simulink library "tqd"  (R2021b)
settings: Solver=VariableStepAuto  StartTime=0.0  StopTime=10.0  RelTol=1e-3
undefined symbols (not defined in the file or in its folder): ATQD_BOSEnBPSPosn_X_kph, ATQD_BOSMap_X_rpm, ATQD_BOSMap_Y_pct, ATQD_CreepBaseTqD_X_kph, ATQD_CreepBaseTqD_Y_Deg, ATQD_CreepBaseTqR_X_kph, ATQD_CreepBaseTqR_Y_Deg, ATQD_CreepBPSDisPosn_X_Deg, ATQD_CreepBPSDisPosnR_X_Deg, ATQD_CreepBPSEnPosn_X_Deg, ATQD_CreepBPSEnPosnR_X_Deg, ATQD_CreepDeltaTq_X_kph, ATQD_CreepIterm_X_kph, ATQD_CreepIterm_Y_kph, ATQD_CreepItermMaxLimit_X_pct, ATQD_CreepPreloadTime_X_kph, ATQD_CreepPreloadTq_X_kph, ATQD_CreepPreloadTq_Y_s, ATQD_CreepProtTq_X_Deg, ATQD_CreepPterm_X_kph, ATQD_ECOTqMapD_X_rpm, ATQD_ECOTqMapD_Y_pct, ATQD_NL1TqMapD_X_rpm, ATQD_NL1TqMapD_Y_pct, ATQD_NRMRrEDUSpRat_X_rpm, ATQD_NRMRrEDUSpRat_Y_Nm, ATQD_PedalMapClimbUpLim_X_rpm, ATQD_PedalMapClimbUpLim_Y_Deg, ATQD_PreLoadTq_X_s, ATQD_SL1TqMapD_X_rpm, ATQD_SL1TqMapD_Y_pct, ATQD_WhlTqCapMotGain_X_pct, ATQD_WhlTqCapMotGain_Y_mV, ENUM_ACCPEDALLOWSW_LOWIDLE, ENUM_ACCPEDALLOWSW_NOIDLE, ENUM_CHRGPLUGSTA_NONE, ENUM_CRASHSTATE_NOCRASH, ENUM_DCDCFAULTSTA_WORKING, ENUM_DRIVEMODE_ECO, ENUM_DRIVEMODE_NRM, ENUM_DRIVEMODE_SPORT, ENUM_DRIVETRAIN_AWD, ENUM_DRIVETRAIN_FWD, ENUM_DRIVETRAIN_RWD, ENUM_EBSBRKSW_PRESSED, ENUM_EBSTORQUERWQ_LIMIT, ENUM_EBSTORQUERWQ_TORQUE, ENUM_EMTRQMODE_ACCL, ENUM_EMTRQMODE_BRAKING, ENUM_EMTRQMODE_COASTING, ENUM_EPBERROR_NORMAL, ENUM_EPBSTA_APPLIED, ENUM_EPBSTA_RELEASED, ENUM_EPBSTA_UNKNOWN, ENUM_EPBSTARAW_NOTSET, ENUM_EPBSTARAW_SET, ENUM_GEARACTUALPOSN_D, ENUM_GEARACTUALPOSN_N, ENUM_GEARACTUALPOSN_P, ENUM_GEARACTUALPOSN_R ... (+201)
libraries: hcu_lib x19, simulink x12
(part 5 of 6)

== system tqd/TQD/TorqueDemand/TorqueModule/AvaliableTqLimit/TorqueCapacityCalcalation ==
  VTQD_FrShaftSpd_rpm : Inport
  VTQD_RrShaftSpd_rpm : Inport  Port=2
  VINP_HVBPwrAvailDchrg_kw : Inport  Port=3
  VINP_HVBPwrAvailChrg_kw : Inport  Port=4
  KTQD_FrBatapCont_factor : Inport  Port=5
  KTQD_RrBatapCont_factor : Inport  Port=6
  VTQD_FrEDUSpRat_cmd : Inport  Port=7
  VTQD_RrEDUSpRat_rat : Inport  Port=8
  VINP_HVBCellVoltMax_mV : Inport  Port=9
  VINP_HVBCellVoltMin_mV : Inport  Port=10
  VINP_HVBSOH_pct : Inport  Port=11
  VTQD_GearActualPosn_enum : Inport  Port=12
  CapacityDistribution : Subsystem
  Constant19 : Constant  Value=MINUSONE_FLOAT
  Constant2 : Constant  Value=ENUM_GEARACTUALPOSN_R
  Data Type Conversion{,1..3} (4 alike) : DataTypeConversion  OutDataTypeStr=single
  Demux : Demux
  Equal : RelationalOperator  Operator===  OutDataTypeStr=boolean  RndMeth=Simplest
  Generation : Subsystem
  Motoring : Subsystem
  Mux : Mux
  Mux1 : Mux
  Product : Product
  Switch : Switch  Criteria=u2 > Threshold
  TMAvailablePwr_Calculation : Subsystem
  VTQD_WhlTqCapGenFr_Nm : Outport
  VTQD_WhlTqCapGenRr_Nm : Outport  Port=2
  VTQD_ActTqCapPosFr_Nm : Outport  Port=3
  VTQD_ActTqCapPosRr_Nm : Outport  Port=4
  VTQD_ActTqCapNegFr_Nm : Outport  Port=5
  VTQD_ActTqCapNegRr_Nm : Outport  Port=6
  wires:
  [VTQD_TMPwrAvailDchrg_kW] -> CapacityDistribution/3(VTQD_TMPwrAvailDchrg_kW)
  TMAvailablePwr_Calculation/1(VTQD_TMPwrAvailDchrg_kW) -> [VTQD_TMPwrAvailDchrg_kW]
  [VINP_HVBPwrAvailDchrg_kw] -> TMAvailablePwr_Calculation/1(VINP_HVBPwrAvailDchrg_kw)
  Motoring/2(VTQD_WhlTqCapMotRr_Nm) -> [VTQD_WhlTqCapMotRr_Nm]
  [VTQD_RrEDUSpRat_rat] -> CapacityDistribution/2(VTQD_RrEDUSpRat_rat)
  [VTQD_FrEDUSpRat_rat] -> CapacityDistribution/1(VTQD_FrEDUSpRat_cmd)
  CapacityDistribution/4(VTQD_RrHVBPwrAvailChrg_kw) -> [VTQD_RrHVBPwrAvailChrg_kw]
  CapacityDistribution/3(VTQD_FrHVBPwrAvailChrg_kw) -> [VTQD_FrHVBPwrAvailChrg_kw]
  CapacityDistribution/2(VTQD_RrHVBPwrAvailDchrg_kw) -> [VTQD_RrHVBPwrAvailDchrg_kw]
  CapacityDistribution/1(VTQD_FrHVBPwrAvailDchrg_kw) -> [VTQD_FrHVBPwrAvailDchrg_kw]
  [VINP_HVBPwrAvailChrg_kw] -> CapacityDistribution/4(VINP_HVBPwrAvailChrg_kw)
  [VTQD_RrHVBPwrAvailChrg_kw] -> Generation/4(VTQD_RrHVBPwrAvailChrg_kw)
  [KTQD_RrBatapCont_factor] -> Generation/6(KTQD_RrBatapCont_factor)
  [VTQD_FrShaftSpd_rpm] -> Generation/1(VTQD_FrShaftSpd_rpm)
  [VTQD_FrHVBPwrAvailChrg_kw] -> Generation/3(VTQD_FrHVBPwrAvailChrg_kw)
  [VTQD_RrShaftSpd_rpm] -> Generation/2(VTQD_RrShaftSpd_rpm)
  [KTQD_FrBatapCont_factor] -> Generation/5(KTQD_FrBatapCont_factor)
  Generation/1(VTQD_WhlTqCapGenFr_Nm) -> [VTQD_WhlTqCapGenFr_Nm], VTQD_WhlTqCapGenFr_Nm/1
  Generation/2(VTQD_WhlTqCapGenRr_Nm) -> [VTQD_WhlTqCapGenRr_Nm], VTQD_WhlTqCapGenRr_Nm/1
  [VTQD_RrHVBPwrAvailDchrg_kw] -> Motoring/4(VTQD_RrHVBPwrAvailDchrg_kw)
  [VTQD_FrHVBPwrAvailDchrg_kw] -> Motoring/3(VTQD_FrHVBPwrAvailDchrg_kw)
  [KTQD_RrBatapCont_factor] -> Motoring/6(KTQD_RrBatapCont_factor)
  VTQD_RrEDUSpRat_rat/1 -> [VTQD_RrEDUSpRat_rat]
  VTQD_FrEDUSpRat_cmd/1 -> [VTQD_FrEDUSpRat_rat]
  KTQD_RrBatapCont_factor/1 -> [KTQD_RrBatapCont_factor]
  [VTQD_RrShaftSpd_rpm] -> Motoring/2(VTQD_RrShaftSpd_rpm)
  VTQD_RrShaftSpd_rpm/1 -> [VTQD_RrShaftSpd_rpm]
  VTQD_FrShaftSpd_rpm/1 -> [VTQD_FrShaftSpd_rpm]
  VINP_HVBPwrAvailChrg_kw/1 -> [VINP_HVBPwrAvailChrg_kw]
  VINP_HVBPwrAvailDchrg_kw/1 -> [VINP_HVBPwrAvailDchrg_kw]
  KTQD_FrBatapCont_factor/1 -> [KTQD_FrBatapCont_factor]
  [VTQD_FrShaftSpd_rpm] -> Motoring/1(VTQD_FrShaftSpd_rpm)
  Motoring/1(VTQD_WhlTqCapMotFr_Nm) -> [VTQD_WhlTqCapMotFr_Nm]
  [KTQD_FrBatapCont_factor] -> Motoring/5(KTQD_FrBatapCont_factor)
  VINP_HVBSOH_pct/1 -> [VINP_HVBSOH_pct]
  VINP_HVBCellVoltMin_mV/1 -> [VINP_HVBCellVoltMin_mV]
  VINP_HVBCellVoltMax_mV/1 -> [VINP_HVBCellVoltMax_mV]
  [VINP_HVBSOH_pct] -> Motoring/9(VINP_HVBSOH_pct)
  [VINP_HVBCellVoltMin_mV] -> Motoring/8(VINP_HVBCellVoltMin_mV)
  [VINP_HVBCellVoltMax_mV] -> Motoring/7(VINP_HVBCellVoltMax_mV)
  VTQD_GearActualPosn_enum/1 -> [VTQD_GearActualPosn_enum]
  [VTQD_GearActualPosn_enum] -> Equal/1
  Constant2/1 -> Equal/2
  Equal/1 -> Switch/2
  Mux/1 -> Product/1
  Product/1 -> Switch/1
  Constant19/1 -> Product/2
  Mux1/1 -> Switch/3
  [VTQD_WhlTqCapMotFr_Nm] -> Mux1/1
  [VTQD_WhlTqCapMotRr_Nm] -> Mux1/2
  [VTQD_WhlTqCapGenFr_Nm] -> Mux1/3
  [VTQD_WhlTqCapGenRr_Nm] -> Mux1/4
  Switch/1 -> Demux/1
  [VTQD_WhlTqCapGenFr_Nm] -> Mux/1
  [VTQD_WhlTqCapGenRr_Nm] -> Mux/2
  [VTQD_WhlTqCapMotFr_Nm] -> Mux/3
  [VTQD_WhlTqCapMotRr_Nm] -> Mux/4
  Demux/1 -> Data Type Conversion/1
  Data Type Conversion/1 -> VTQD_ActTqCapPosFr_Nm/1  "VTQD_ActTqCapPosFr_Nm"
  Demux/2 -> Data Type Conversion1/1
  Data Type Conversion1/1 -> VTQD_ActTqCapPosRr_Nm/1  "VTQD_ActTqCapPosRr_Nm"
  Demux/3 -> Data Type Conversion2/1
  Data Type Conversion2/1 -> VTQD_ActTqCapNegFr_Nm/1  "VTQD_ActTqCapNegFr_Nm"
  Demux/4 -> Data Type Conversion3/1
  Data Type Conversion3/1 -> VTQD_ActTqCapNegRr_Nm/1  "VTQD_ActTqCapNegRr_Nm"

== system tqd/TQD/TorqueDemand/TorqueModule/DriverWhlTqDem/BOS ==
  VTQD_ActBPSPosn_pct : Inport
  VTQD_TqTargetShaftSpd_rpm : Inport  Port=2
  VTQD_VehActSpd_kph : Inport  Port=3
  VTQD_PedalMapWhlTq_Nm : Inport  Port=4
  VTQD_CreepBaseTqR_Nm : Inport  Port=5
  VTQD_CreepBaseTqD_Nm : Inport  Port=6
  VTQD_GearActualPosn_enum : Inport  Port=7
  VTQD_LowIdleAccPedal_flg : Inport  Port=8
  VTQD_HighBPSPosn_flg : Inport  Port=9
  VTQD_BrkSwSta_flg : Inport  Port=10
  AND : Logic  Inputs=3  AllPortsSameDT=off  OutDataTypeStr=boolean
  AND1 : Logic  AllPortsSameDT=off  OutDataTypeStr=boolean
  AND2 : Logic  AllPortsSameDT=off  OutDataTypeStr=boolean
  Constant1 : Constant  Value=KTQD_BOSEnPedalTq_Nm
  Constant18 : Constant  Value=ZERO_FLOAT
  Constant20 : Constant  Value=ENUM_GEARACTUALPOSN_R
  Constant3 : Constant  Value=ONE_PERCENT
  Detect Change : simulink/Logic and Bit Operations/Detect Change  vinit=0  OutDataTypeStr=boolean
  Equal10 : RelationalOperator  Operator===  OutDataTypeStr=boolean  RndMeth=Simplest
  MTQD_BOSEnBPSPosn_Y_pct : Lookup_n-D  NumberOfTableDimensions=1  BreakpointsForDimension1=ATQD_BOSEnBPSPosn_X_kph  Table=MTQD_BOSEnBPSPosn_Y_pct  InternalRulePriority=Speed  RndMeth=Simplest  InputSameDT=on
  MTQD_BOSMap_Z_pct : Lookup_n-D  BreakpointsForDimension1=ATQD_BOSMap_Y_pct  BreakpointsForDimension2=ATQD_BOSMap_X_rpm  Table=MTQD_BOSMap_Z_pct  ExtrapMethod=Clip  InternalRulePriority=Speed  RndMeth=Simplest  InputSameDT=on
      settings: InputPortMap=u0,u1
  Max : MinMax  Function=max  Inputs=2
  NOT1 : Logic  Operator=NOT  AllPortsSameDT=off  OutDataTypeStr=boolean
  NOT2 : Logic  Operator=NOT  AllPortsSameDT=off  OutDataTypeStr=boolean
  NOT3 : Logic  Operator=NOT  AllPortsSameDT=off  OutDataTypeStr=boolean
  OR : Logic  Operator=OR  Inputs=3  AllPortsSameDT=off  OutDataTypeStr=boolean
  OR1 : Logic  Operator=OR  AllPortsSameDT=off  OutDataTypeStr=boolean
  Product1 : Product  RndMeth=Zero
  Product2 : Product  RndMeth=Zero
  Product3 : Product  RndMeth=Zero
  Relational Operator : RelationalOperator  Operator=>  OutDataTypeStr=boolean  RndMeth=Simplest
  Relational Operator1 : RelationalOperator  Operator=>  OutDataTypeStr=boolean  RndMeth=Simplest
  Relational Operator2 : RelationalOperator  OutDataTypeStr=boolean  RndMeth=Simplest
  Relational Operator5 : RelationalOperator  Operator=>  OutDataTypeStr=boolean  RndMeth=Simplest
  SR_Latch : hcu_lib/Basic_Blocks/SR_Latch
  Switch7 : Switch  Criteria=u2 > Threshold
  Switch8 : Switch  Criteria=u2 > Threshold
  VTQD_BOSEnable_flg : Outport
  VTQD_BOSTq_Nm : Outport  Port=2
  wires:
  VTQD_TqTargetShaftSpd_rpm/1 -> [VTQD_TqTargetShaftSpd_rpm]
  [VTQD_ActBPSPosn_pct] -> MTQD_BOSMap_Z_pct/1
  [VTQD_TqTargetShaftSpd_rpm] -> MTQD_BOSMap_Z_pct/2
  Constant3/1 -> Product1/2
  Product1/1 -> [VTQD_BOSReduction_gain]  "VTQD_BOSReduction_gain"
  MTQD_BOSMap_Z_pct/1 -> Product1/1
  VTQD_ActBPSPosn_pct/1 -> [VTQD_ActBPSPosn_pct]
  Relational Operator/1 -> AND/1
  VTQD_VehActSpd_kph/1 -> [VTQD_VehActSpd_kph]
  [VTQD_VehActSpd_kph] -> MTQD_BOSEnBPSPosn_Y_pct/1
  MTQD_BOSEnBPSPosn_Y_pct/1 -> Relational Operator/2  "VTQD_BOSEnBPSPosn_pct"
  [VTQD_ActBPSPosn_pct] -> Relational Operator/1
  VTQD_PedalMapWhlTq_Nm/1 -> [VTQD_PedalMapWhlTq_Nm]
  Relational Operator1/1 -> AND/2
  [VTQD_PedalMapWhlTq_Nm] -> Relational Operator1/1
  Constant1/1 -> Relational Operator1/2
  [VTQD_PedalMapWhlTq_Nm] -> Product2/1
  [VTQD_BOSReduction_gain] -> Product2/2
  Product3/1 -> Max/2
  Switch8/1 -> VTQD_BOSTq_Nm/1, [VTQD_BOSTq_Nm]  "VTQD_BOSTq_Nm"
  [VTQD_CreepBaseTqR_Nm] -> Switch7/1
  Max/1 -> Switch8/1
  Product2/1 -> Switch8/3
  Equal10/1 -> Switch7/2
  [VTQD_PedalMapWhlTq_Nm] -> Product3/1
  [VTQD_BOSReduction_gain] -> Product3/2
  [VTQD_GearActualPosn_enum] -> Equal10/1
  Relational Operator5/1 -> Switch8/2
  Constant20/1 -> Equal10/2
  Switch7/1 -> Max/1
  Constant18/1 -> Relational Operator5/2
  [VTQD_CreepBaseTqD_Nm] -> Switch7/3
  VTQD_CreepBaseTqD_Nm/1 -> [VTQD_CreepBaseTqD_Nm]
  VTQD_CreepBaseTqR_Nm/1 -> [VTQD_CreepBaseTqR_Nm]
  VTQD_GearActualPosn_enum/1 -> [VTQD_GearActualPosn_enum]
  [VTQD_BOSReduction_gain] -> Relational Operator5/1
  AND/1 -> SR_Latch/1, NOT1/1
  SR_Latch/1 -> VTQD_BOSEnable_flg/1  "VTQD_BOSEnable_flg"
  NOT1/1 -> AND1/1
  [VTQD_BOSTq_Nm] -> Relational Operator2/2
  [VTQD_PedalMapWhlTq_Nm] -> Relational Operator2/1
  VTQD_LowIdleAccPedal_flg/1 -> [VTQD_LowIdleAccPedal_flg]
  [VTQD_LowIdleAccPedal_flg] -> NOT2/1
  NOT2/1 -> AND/3
  [VTQD_BrkSwSta_flg] -> NOT3/1
  AND2/1 -> OR/3
  [VTQD_GearActualPosn_enum] -> Detect Change/1
  [VTQD_HighBPSPosn_flg] -> OR/2
  NOT3/1 -> AND2/2
  [VTQD_LowIdleAccPedal_flg] -> AND2/1
  OR/1 -> AND1/2
  Detect Change/1 -> OR1/2
  Relational Operator2/1 -> OR/1
  AND1/1 -> OR1/1
  OR1/1 -> SR_Latch/2
  VTQD_BrkSwSta_flg/1 -> [VTQD_BrkSwSta_flg]
  VTQD_HighBPSPosn_flg/1 -> [VTQD_HighBPSPosn_flg]

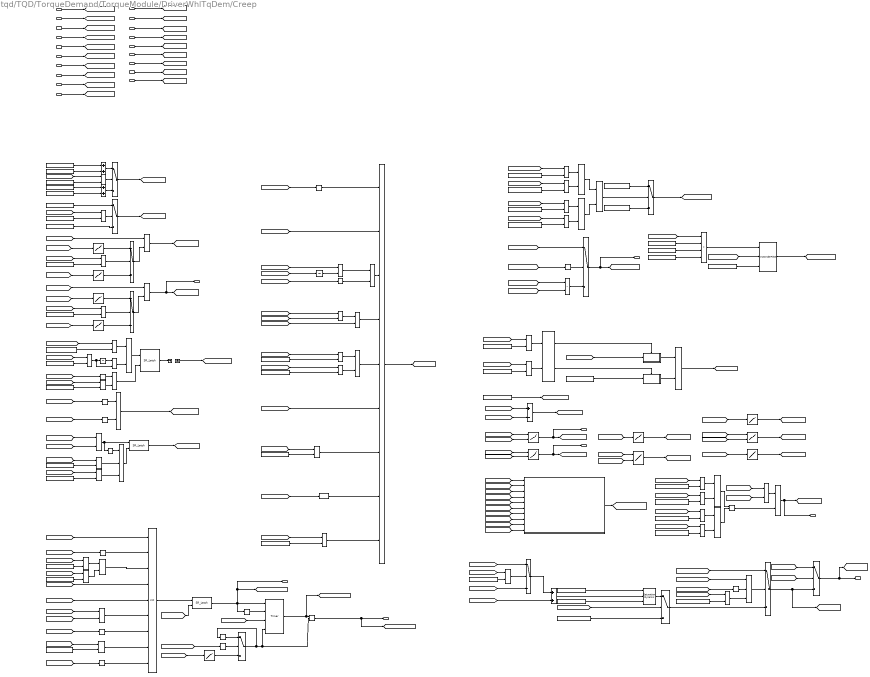
== system tqd/TQD/TorqueDemand/TorqueModule/DriverWhlTqDem/Creep ==
  note: Creep Enable Judgement
  note: Vehicle Actual Speed Calculation
  note: Creep Wheel Torque Demand Calculation
  VTQD_CreepON_flg : Inport
  VTQD_GearActualPosn_enum : Inport  Port=2
  VTQD_LowIdleAccPedal_flg : Inport  Port=3
  VINP_VehSpeed_kph : Inport  Port=4
  VTQD_TMRotateDirction_enum : Inport  Port=5
  VTQD_RegenMode_enum : Inport  Port=6
  VTQD_ActBPSPosn_pct : Inport  Port=7
  VTQD_PedalMapWhlTq_Nm : Inport  Port=8
  VINP_RrRBCActive_flg : Inport  Port=9
  VINP_FrRBCActive_flg : Inport  Port=10
  task_time_s : Inport  Port=11
  VTQD_RDCActive_enum : Inport  Port=12
  " VINP_FrEDURealTMTq_Nm" : Inport  Port=13
  VINP_RrEDURealTMTq_Nm : Inport  Port=14
  VTQD_PreLoadPreEn_flg : Inport  Port=15
  VVMC_EstSlope_Deg : Inport  Port=16
  VPMM_PwrSta_enum : Inport  Port=17
  VTQD_TqTargetShaftSpd_rpm : Inport  Port=18
  VINP_EPBSta_enum : Inport  Port=19
  AND{1..2,4,6..7} (5 alike) : Logic  AllPortsSameDT=off  OutDataTypeStr=boolean
  AND3 : Logic  Inputs=3  AllPortsSameDT=off  OutDataTypeStr=boolean
  AND8 : Logic  Inputs=3  AllPortsSameDT=off  OutDataTypeStr=boolean
  Add : Sum  Inputs=+-
  Add1 : Sum
  Add2 : Sum
  Add4 : Sum
  Constant10 : Constant  Value=KTQD_CreepTargetSpdR_kph
  Constant{3,11..12,21} (4 alike) : Constant  Value=ENUM_GEARACTUALPOSN_D
  Constant13 : Constant  Value=KTQD_CreepEnableSpd_kph
  Constant14 : Constant  Value=RPM2RADPS
  Constant15 : Constant  Value=ZERO_FLOAT
  Constant16 : Constant  Value=KTQD_TireRadius_m
  Constant17 : Constant  Value=ENUM_RDCACTSTA_NOREQUEST
  Constant19 : Constant  Value=MPS2KPH
  Constant{2,9,20,31,35..36,38,42..44} (10 alike) : Constant  Value=ENUM_GEARACTUALPOSN_R
  Constant22 : Constant  Value=KTQD_CreepLowLimitTq_Nm
  Constant23 : Constant  Value=KTQD_CreepPrLoadEnSpd_kph
  Constant24 : Constant  Value=ENUM_RDCACTSTA_NOREQUEST
  Constant26 : Constant  Value=KTQD_CreepDisableSpdofst_kph
  Constant27 : Constant  Value=KTQD_CreepEnableSpdR_kph
  Constant28 : Constant  Value=KTQD_CreepDisableSpdofstR_kph
  Constant29 : Constant  Value=KTQD_CreepEnableSpdR_kph
  Constant30 : Constant  Value=ENUM_TMROTATEDIRECTACT_REVERSE  OutDataTypeStr=Inherit: Inherit via back propagation
  Constant32 : Constant  Value=ENUM_TMROTATEDIRECTACT_FORWARD  OutDataTypeStr=Inherit: Inherit via back propagation
  Constant33 : Constant  Value=KTQD_VehActSpdNegGain_gain
  Constant34 : Constant  Value=KTQD_VehActSpdPosGain_gain
  Constant37 : Constant  Value=ENUM_TMROTATEDIRECTACT_REVERSE  OutDataTypeStr=Inherit: Inherit via back propagation
  Constant39 : Constant  Value=ENUM_TMROTATEDIRECTACT_FORWARD  OutDataTypeStr=Inherit: Inherit via back propagation
  Constant4 : Constant  Value=ENUM_REGENLEVEL_OPD
  Constant40 : Constant  Value=KTQD_RBCCreepRecTq_Nm
  Constant41 : Constant  Value=KTQD_RBCCreepRecTq_Nm
  Constant45 : Constant  Value=ENUM_POWERSTA_READY
  Constant46 : Constant  Value=KTQD_CreepEnableSpd_kph
  Constant47 : Constant  Value=KTQD_RPM2VehSpdTs_c
  Constant49 : Constant  Value=KTQD_CreepTargetSpdD_kph
  Constant55 : Constant  Value=ENUM_EPBSTA_APPLIED  OutDataTypeStr=uint8
  Constant57 : Constant  Value=KTQD_CreepUpLimitTq_Nm
  Constant6 : Constant  Value=ENUM_GEARACTUALPOSN_P
  Constant7 : Constant  Value=ENUM_GEARACTUALPOSN_N
  Delay : Delay  DelayLength=1
  Delay1 : Delay  DelayLength=1
  Detect Change : simulink/Logic and Bit Operations/Detect Change  vinit=0  OutDataTypeStr=boolean
  Equal{,1..4,6..8,10,12..14,16,21..30,34} (24 alike) : RelationalOperator  Operator===  OutDataTypeStr=boolean  RndMeth=Simplest
  Equal17 : RelationalOperator  Operator=<=  OutDataTypeStr=boolean  RndMeth=Simplest
  Equal18 : RelationalOperator  Operator=~=  OutDataTypeStr=boolean  RndMeth=Simplest
  Equal5 : RelationalOperator  Operator=<=  OutDataTypeStr=boolean  RndMeth=Simplest
  Equal9 : RelationalOperator  Operator=<=  OutDataTypeStr=boolean  RndMeth=Simplest
  FirstOrderFilter : hcu_lib/Basic_Blocks/FirstOrderFilter
  GreaterThan : RelationalOperator  Operator=>  OutDataTypeStr=boolean  RndMeth=Simplest
  GreaterThan1 : RelationalOperator  Operator=>  OutDataTypeStr=boolean  RndMeth=Simplest
  GreaterThan2 : RelationalOperator  OutDataTypeStr=boolean  RndMeth=Simplest
  GreaterThan3 : RelationalOperator  Operator=>  OutDataTypeStr=boolean  RndMeth=Simplest
  Ground2 : Ground
  If : If  NumInputs=2  IfExpression=u1 ~= 0  ElseIfExpressions=u2 ~= 0  ShowElse=off
  If Action Subsystem : Subsystem  TreatAsAtomicUnit=on
  If Action Subsystem1 : Subsystem  TreatAsAtomicUnit=on
  LiuzgSwitch1 : Switch  Criteria=u2 ~= 0
      settings: AttributesFormatString=<%<Criteria>>
  Logical Operator{,2,4,6} (4 alike) : Logic  AllPortsSameDT=off  OutDataTypeStr=boolean
  Logical Operator1 : Logic  Operator=OR  AllPortsSameDT=off  OutDataTypeStr=boolean
  Logical Operator3 : Logic  Inputs=9  AllPortsSameDT=off  OutDataTypeStr=boolean
  Logical Operator5 : Logic  Operator=OR  AllPortsSameDT=off  OutDataTypeStr=boolean
  MTQD_CreepBPSDisPosnR_Y_pct : Lookup_n-D  NumberOfTableDimensions=1  BreakpointsForDimension1=ATQD_CreepBPSDisPosnR_X_Deg  Table=MTQD_CreepBPSDisPosnR_Y_pct  ExtrapMethod=Clip  InternalRulePriority=Speed  RndMeth=Simplest  InputSameDT=on
  MTQD_CreepBPSDisPosn_Y_pct : Lookup_n-D  NumberOfTableDimensions=1  BreakpointsForDimension1=ATQD_CreepBPSDisPosn_X_Deg  Table=MTQD_CreepBPSDisPosn_Y_pct  ExtrapMethod=Clip  InternalRulePriority=Speed  RndMeth=Simplest  InputSameDT=on
  MTQD_CreepBPSEnPosnR_Y_pct : Lookup_n-D  NumberOfTableDimensions=1  BreakpointsForDimension1=ATQD_CreepBPSEnPosnR_X_Deg  Table=MTQD_CreepBPSEnPosnR_Y_pct  ExtrapMethod=Clip  InternalRulePriority=Speed  RndMeth=Simplest  InputSameDT=on
  MTQD_CreepBPSEnPosn_Y_pct : Lookup_n-D  NumberOfTableDimensions=1  BreakpointsForDimension1=ATQD_CreepBPSEnPosn_X_Deg  Table=MTQD_CreepBPSEnPosn_Y_pct  ExtrapMethod=Clip  InternalRulePriority=Speed  RndMeth=Simplest  InputSameDT=on
  MTQD_CreepBaseTqD_Z_Nm : Lookup_n-D  BreakpointsForDimension1=ATQD_CreepBaseTqD_Y_Deg  BreakpointsForDimension2=ATQD_CreepBaseTqD_X_kph  Table=MTQD_CreepBaseTqD_Z_Nm  ExtrapMethod=Clip  InternalRulePriority=Speed  RndMeth=Simplest  InputSameDT=on
      settings: InputPortMap=u0,u1
  MTQD_CreepBaseTqR_Z_Nm : Lookup_n-D  BreakpointsForDimension1=ATQD_CreepBaseTqR_Y_Deg  BreakpointsForDimension2=ATQD_CreepBaseTqR_X_kph  Table=MTQD_CreepBaseTqR_Z_Nm  ExtrapMethod=Clip  InternalRulePriority=Speed  RndMeth=Simplest  InputSameDT=on
      settings: InputPortMap=u0,u1
  MTQD_CreepDeltaTq_Y_Nm : Lookup_n-D  NumberOfTableDimensions=1  BreakpointsForDimension1=ATQD_CreepDeltaTq_X_kph  Table=MTQD_CreepDeltaTq_Y_Nm  ExtrapMethod=Clip  InternalRulePriority=Speed  RndMeth=Simplest  InputSameDT=on
  MTQD_CreepIterm_Z_Nm : Lookup_n-D  BreakpointsForDimension1=ATQD_CreepIterm_Y_kph  BreakpointsForDimension2=ATQD_CreepIterm_X_kph  Table=MTQD_CreepIterm_Z_Nm  ExtrapMethod=Clip  InternalRulePriority=Speed  RndMeth=Simplest  InputSameDT=on
      settings: InputPortMap=u0,u1
  MTQD_CreepPrelaodTq_Z_Nm : Lookup_n-D  BreakpointsForDimension1=ATQD_CreepPreloadTq_Y_s  BreakpointsForDimension2=ATQD_CreepPreloadTq_X_kph  Table=MTQD_CreepPreloadTq_Z_Nm  ExtrapMethod=Clip  InternalRulePriority=Speed  RndMeth=Simplest  InputSameDT=on
      settings: InputPortMap=u0,u1
  MTQD_CreepPreloadTime_Y_s : Lookup_n-D  NumberOfTableDimensions=1  BreakpointsForDimension1=ATQD_CreepPreloadTime_X_kph  Table=MTQD_CreepPreloadTime_Y_s  ExtrapMethod=Clip  InternalRulePriority=Speed  RndMeth=Simplest  InputSameDT=on
  MTQD_CreepProtTq_Y_Nm : Lookup_n-D  NumberOfTableDimensions=1  BreakpointsForDimension1=ATQD_CreepProtTq_X_Deg  Table=MTQD_CreepProtTq_Y_Nm  ExtrapMethod=Clip  InternalRulePriority=Speed  RndMeth=Simplest  InputSameDT=on
  MTQD_CreepPterm_Y_c : Lookup_n-D  NumberOfTableDimensions=1  BreakpointsForDimension1=ATQD_CreepPterm_X_kph  Table=MTQD_CreepPterm_Y_Nm  ExtrapMethod=Clip  InternalRulePriority=Speed  RndMeth=Simplest  InputSameDT=on
  Merge : Merge
  NOT{,1..2,4,6..8,10..13} (11 alike) : Logic  Operator=NOT  AllPortsSameDT=off  OutDataTypeStr=boolean
  OR{,2,6..7} (4 alike) : Logic  Operator=OR  AllPortsSameDT=off  OutDataTypeStr=boolean
  OR1 : Logic  Operator=OR  Inputs=9  AllPortsSameDT=off  OutDataTypeStr=boolean
  Product : Product
  Product1 : Product  Inputs=4
  Relational Operator : RelationalOperator  OutDataTypeStr=boolean  RndMeth=Simplest
  Relational Operator2 : RelationalOperator  Operator=>  OutDataTypeStr=boolean  RndMeth=Simplest
  Relational Operator3 : RelationalOperator  Operator=>  OutDataTypeStr=boolean  RndMeth=Simplest
  Relational Operator4 : RelationalOperator  Operator=>  OutDataTypeStr=boolean  RndMeth=Simplest
  Relay1 : Relay  OnSwitchValue=KTQD_CreepDisVehSpd_kph  OffSwitchValue=KTQD_CreepEnVehSpd_kph  OnOutputValue=0  OffOutputValue=1  OutDataTypeStr=boolean
  SR_Latch : hcu_lib/Basic_Blocks/SR_Latch
  SR_Latch1 : hcu_lib/Basic_Blocks/SR_Latch
  SR_Latch3 : hcu_lib/Basic_Blocks/SR_Latch
  Saturation Dynamic : simulink/Discontinuities/Saturation Dynamic  OutMin=[]  OutMax=[]  OutDataTypeStr=Inherit: Same as second input  OutDataType=fixdt(1, 16)  OutScaling=2^-10  DoSatur=off
  Switch{,3..4,7} (4 alike) : Switch  Criteria=u2 ~= 0
  Switch Case Action Subsystem : Subsystem  TreatAsAtomicUnit=on
  Switch{5..6,8..11} (6 alike) : Switch  Criteria=u2 > Threshold
  Terminator3 : Terminator
  Timer : hcu_lib/Basic_Blocks/Timer
  Unit Delay : UnitDelay  SampleTime=-1  HasFrameUpgradeWarning=on
  Unit Delay1 : UnitDelay  SampleTime=-1  HasFrameUpgradeWarning=on
  VTQD_CreepEnable_flg : Outport
  VTQD_CreepWhlTqDem_Nm : Outport  Port=2
  VTQD_CreepPrLoadEnable_flg : Outport  Port=3
  VTQD_CreepProtTqEn_flg : Outport  Port=4
  VTQD_VehActSpd_kph : Outport  Port=5
  VTQD_CreepBaseTqD_Nm : Outport  Port=6
  VTQD_CreepBaseTqR_Nm : Outport  Port=7
  VTQD_HighBPSPosn_flg : Outport  Port=8
  wires:
  [VTQD_CreepTotalOfstTq_Nm] -> Add2/2
  If Action Subsystem1/1(VTQD_CreepTotalOfstTq_Nm) -> [VTQD_CreepTotalOfstTq_Nm]  "VTQD_CreepTotalOfstTq_Nm"
  [VTQD_ActBPSPosn_pct] -> If Action Subsystem1/6(VTQD_ActBPSPosn_pct)
  [task_time_s] -> If Action Subsystem1/7(task_time_s)
  [VTQD_CreepDeltaTq_Nm] -> If Action Subsystem1/5(VTQD_CreepDeltaTq_Nm)
  task_time_s/1 -> [task_time_s]
  [VTQD_CreepIterm_c] -> If Action Subsystem1/4(VTQD_CreepIterm_c)
  [VTQD_CreepPterm_c] -> If Action Subsystem1/3(VTQD_CreepPterm_c)
  [VTQD_CreepErrSpd_kph] -> If Action Subsystem1/2(VTQD_CreepErrSpd_kph)
  [VTQD_ActBPSPosnInRange_flg] -> If Action Subsystem1/1(VTQD_ActBPSPosnInRange_flg)
  AND6/1 -> [VTQD_ActBPSPosnInRange_flg]  "VTQD_ActBPSPosnInRange_flg"
  [VTQD_CreepEnable_flg] -> If Action Subsystem1/9(VTQD_CreepEnable_flg)
  NOT4/1 -> Logical Operator3/2
  [VTQD_OPDOn2Off_flg] -> NOT4/1
  NOT/1 -> Logical Operator3/7
  Merge/1 -> [VTQD_CreepFinalSpd_kph]  "VTQD_CreepFinalSpd_kph"
  Switch Case Action Subsystem/1(Out1) -> Merge/2
  If Action Subsystem/1(Out1) -> Merge/1
  If/2 -> Switch Case Action Subsystem/Action
  If/1 -> If Action Subsystem/Action
  Equal12/1 -> If/2
  Constant2/1 -> Equal12/2
  [VTQD_GearActualPosn_enum] -> Equal12/1
  Equal13/1 -> If/1
  Constant12/1 -> Equal13/2
  [VTQD_GearActualPosn_enum] -> Equal13/1
  [VTQD_HighBPSPosn_flg] -> OR1/2
  [VTQD_RBCActive_flg] -> NOT/1
  [VTQD_CreepEnSpd_kph] -> Equal9/2
  VINP_FrRBCActive_flg/1 -> [VINP_FrRBCActive_flg]
  VINP_RrRBCActive_flg/1 -> [VINP_RrRBCActive_flg]
  OR1/1 -> [VTQD_CreepDisable_flg]  "VTQD_CreepDisable_flg"
  [VTQD_CreepDisable_flg] -> SR_Latch/2
  [VTQD_CreepON_flg] -> NOT2/1
  Equal10/1 -> OR/2
  Equal6/1 -> OR/1
  Constant7/1 -> Equal10/2
  [VTQD_GearActualPosn_enum] -> Equal10/1
  Constant6/1 -> Equal6/2
  [VTQD_GearActualPosn_enum] -> Equal6/1
  [VTQD_LowIdleAccPedal_flg] -> NOT1/1
  [VTQD_LowIdleAccPedal_flg] -> AND2/2
  GreaterThan1/1 -> AND2/1
  [VTQD_CreepDisSpd_kph] -> GreaterThan1/2
  [VTQD_VehActSpd_kph] -> GreaterThan1/1
  Unit Delay/1 -> GreaterThan/2
  [VTQD_CreepWhlTqDem_Nm] -> Unit Delay/1
  [VTQD_PedalMapWhlTq_Nm] -> GreaterThan/1
  VTQD_PedalMapWhlTq_Nm/1 -> [VTQD_PedalMapWhlTq_Nm]
  [VTQD_LowBPSPosn_flg] -> Logical Operator3/4
  VTQD_ActBPSPosn_pct/1 -> [VTQD_ActBPSPosn_pct]
  Equal7/1 -> Logical Operator5/1
  [VTQD_GearActualPosn_enum] -> Equal8/1
  Equal8/1 -> Logical Operator5/2
  Constant20/1 -> Equal7/2
  Constant21/1 -> Equal8/2
  [VTQD_GearActualPosn_enum] -> Equal7/1
  [VTQD_LowIdleAccPedal_flg] -> Logical Operator3/5
  [VTQD_VehActSpd_kph] -> Equal9/1
  Logical Operator5/1 -> Logical Operator3/3
  Equal9/1 -> Logical Operator3/6
  VTQD_RegenMode_enum/1 -> [VTQD_RegenMode_enum]
  Constant34/1 -> LiuzgSwitch1/3
  Constant33/1 -> LiuzgSwitch1/1
  VTQD_TMRotateDirction_enum/1 -> [VTQD_TMRotateDirction_enum]
  [VTQD_TMRotateDirction_enum] -> Equal1/1
  Constant3/1 -> Equal/2
  Equal/1 -> Logical Operator/1
  [VTQD_GearActualPosn_enum] -> Equal/1
  LiuzgSwitch1/1 -> [VTQD_VehActSpdGain_gain]  "VTQD_VehActSpdGain_gain"
  Equal3/1 -> Logical Operator2/2
  Constant30/1 -> Equal1/2
  Equal1/1 -> Logical Operator/2
  Constant31/1 -> Equal2/2
  Equal2/1 -> Logical Operator2/1
  Logical Operator2/1 -> Logical Operator1/2
  Logical Operator1/1 -> LiuzgSwitch1/2
  Logical Operator/1 -> Logical Operator1/1
  [VTQD_GearActualPosn_enum] -> Equal2/1
  [VTQD_TMRotateDirction_enum] -> Equal3/1
  Constant32/1 -> Equal3/2
  VTQD_LowIdleAccPedal_flg/1 -> [VTQD_LowIdleAccPedal_flg]
  VTQD_CreepON_flg/1 -> [VTQD_CreepON_flg]
  Logical Operator3/1 -> SR_Latch/1
  VTQD_GearActualPosn_enum/1 -> [VTQD_GearActualPosn_enum]
  VINP_VehSpeed_kph/1 -> [VINP_VehSpeed_kph]
  SR_Latch3/1 -> Terminator3/1
  Switch/1 -> Switch4/3
  [VTQD_CreepEnable_flg] -> Switch/2
  Constant15/1 -> Switch/3
  [VTQD_CreepDisable_flg] -> If Action Subsystem1/8(VTQD_CreepDisable_flg)
  [VTQD_CreepTargetSpdD_kph] -> If Action Subsystem/1(In1)
  Constant10/1 -> Switch Case Action Subsystem/1(In1)
  [VTQD_CreepON_flg] -> Logical Operator3/1
  NOT2/1 -> OR1/1
  [VTQD_CreepBaseTqD_Nm] -> Switch3/3
  [VTQD_CreepBaseTqR_Nm] -> Switch3/1
  Switch3/1 -> Add2/1  "VTQD_ActCreepBaseTq_Nm"
  Constant9/1 -> Equal16/2
  [VTQD_GearActualPosn_enum] -> Equal16/1
  Equal16/1 -> Switch3/2
  Timer/1 -> [VTQD_CreepPreloadTime_s], Relational Operator/1  "VTQD_CreepPreloadTime_s"
  [task_time_s] -> Timer/3
  Relational Operator/1 -> [VTQD_CreepEnable_flg], VTQD_CreepEnable_flg/1  "VTQD_CreepEnable_flg"
  SR_Latch/1 -> VTQD_CreepPrLoadEnable_flg/1, [VTQD_CreepPrLoadEnable_flg], NOT8/1, Timer/1  "VTQD_CreepPrLoadEnable_flg"
  NOT8/1 -> Timer/2
  [VTQD_CreepEnable_flg] -> NOT10/1
  NOT10/1 -> AND3/2
  [VTQD_CreepPreloadTq_Nm] -> Switch4/1
  [VTQD_CreepPrLoadEnable_flg] -> AND3/1
  AND3/1 -> Switch4/2
  [VTQD_OPDOn2Off_flg] -> If Action Subsystem1/10(VTQD_OPDOn2Off)
  [VINP_VehSpeed_kph] -> Equal17/1
  Constant23/1 -> Equal17/2
  Equal17/1 -> AND3/3
  AND1/1 -> OR1/3
  AND2/1 -> OR1/4
  VTQD_RDCActive_enum/1 -> [VTQD_RDCActive_enum]
  [VTQD_RDCActive_enum] -> Equal14/1
  Constant17/1 -> Equal14/2
  Constant24/1 -> Equal18/2
  [VTQD_RDCActive_enum] -> Equal18/1
  Equal22/1 -> Switch6/2
  Constant29/1 -> Switch6/1
  Switch6/1 -> [VTQD_CreepEnSpd_kph]  "VTQD_CreepEnSpd_kph"
  Constant36/1 -> Equal22/2
  Switch5/1 -> [VTQD_CreepDisSpd_kph]  "VTQD_CreepDisSpd_kph"
  Constant35/1 -> Equal21/2
  [VTQD_GearActualPosn_enum] -> Equal22/1
  Add1/1 -> Switch5/1
  [VTQD_GearActualPosn_enum] -> Equal21/1
  Equal21/1 -> Switch5/2
  Constant27/1 -> Add1/1
  Add4/1 -> Switch5/3
  Constant13/1 -> Add4/1
  Constant26/1 -> Add4/2
  Constant28/1 -> Add1/2
  AND7/1 -> VTQD_CreepProtTqEn_flg/1, [VTQD_CreepProtTqEn_flg]  "VTQD_CreepProtTqEn_flg"
  Equal25/1 -> Logical Operator6/1
  [VTQD_GearActualPosn_enum] -> Equal25/1
  [VTQD_CreepProtTq_Nm] -> Relational Operator2/1
  Constant38/1 -> Equal25/2
  Relational Operator2/1 -> AND7/1
  [VTQD_CreepActWhlTqDem_Nm] -> Relational Operator2/2
  [VTQD_TMRotateDirction_enum] -> Equal26/1
  Constant39/1 -> Equal26/2
  Logical Operator4/1 -> OR6/1
  [VTQD_GearActualPosn_enum] -> Equal23/1
  [VTQD_TMRotateDirction_enum] -> Equal24/1
  Constant11/1 -> Equal23/2
  Equal23/1 -> Logical Operator4/1
  Equal24/1 -> Logical Operator4/2
  Constant37/1 -> Equal24/2
  OR6/1 -> AND7/2
  Equal26/1 -> Logical Operator6/2
  Logical Operator6/1 -> OR6/2
  Switch4/1 -> [VTQD_CreepActWhlTqDem_Nm], Switch7/3  "VTQD_CreepActWhlTqDem_Nm"
  [VTQD_CreepProtTqEn_flg] -> Switch7/2
  Switch7/1 -> VTQD_CreepWhlTqDem_Nm/1, [VTQD_CreepWhlTqDem_Nm]  "VTQD_CreepWhlTqDem_Nm"
  [VTQD_CreepProtTq_Nm] -> Switch7/1
  Relational Operator4/1 -> AND8/2
  NOT7/1 -> AND8/1
  SR_Latch1/1 -> [VTQD_RBCActive_flg]  "VTQD_RBCActive_flg"
  AND8/1 -> SR_Latch1/2  "VTQD_RBCActiveRec_flg"
  Constant41/1 -> Relational Operator4/2
  OR7/1 -> NOT7/1, SR_Latch1/1
  [VINP_FrEDURealTMTq_Nm] -> Relational Operator4/1
  Constant40/1 -> Relational Operator3/2
  [VINP_RrEDURealTMTq_Nm] -> Relational Operator3/1
  Relational Operator3/1 -> AND8/3
  [VINP_RrRBCActive_flg] -> OR7/1
  [VINP_FrRBCActive_flg] -> OR7/2
  VINP_RrEDURealTMTq_Nm/1 -> [VINP_RrEDURealTMTq_Nm]
  " VINP_FrEDURealTMTq_Nm"/1 -> [VINP_FrEDURealTMTq_Nm]
  Ground2/1 -> [VTQD_OPDOn2Off_flg]  "VTQD_OPDOn2Off_flg"
  VTQD_PreLoadPreEn_flg/1 -> [VTQD_PreLoadPreEn_flg]
  VVMC_EstSlope_Deg/1 -> [VVMC_EstSlope_Deg]
  VPMM_PwrSta_enum/1 -> [VPMM_PwrSta_enum]
  [VPMM_PwrSta_enum] -> Equal30/1
  Equal29/1 -> OR2/2
  [VTQD_GearActualPosn_enum] -> Equal29/1
  Equal4/1 -> GreaterThan3/2, Unit Delay1/1
  Constant4/1 -> Equal4/2
  [VTQD_LowIdleAccPedal_flg] -> NOT6/1
  GreaterThan3/1 -> AND4/2
  Equal30/1 -> AND4/1
  Constant45/1 -> Equal30/2
  Constant44/1 -> Equal29/2
  NOT6/1 -> OR2/1
  [VTQD_RegenMode_enum] -> Equal4/1
  OR2/1 -> SR_Latch3/2
  Unit Delay1/1 -> GreaterThan3/1
  AND4/1 -> SR_Latch3/1
  Constant43/1 -> Equal28/2
  [VVMC_EstSlope_Deg] -> MTQD_CreepBPSDisPosnR_Y_pct/1
  Equal27/1 -> Switch8/2
  MTQD_CreepBPSDisPosn_Y_pct/1 -> Switch9/3  "VTQD_CreepBPSDisPosn_pct"
  [VTQD_ActBPSPosn_pct] -> GreaterThan2/1
  GreaterThan2/1 -> VTQD_HighBPSPosn_flg/1, [VTQD_HighBPSPosn_flg]  "VTQD_HighBPSPosn_flg"
  Switch9/1 -> GreaterThan2/2
  Equal5/1 -> [VTQD_LowBPSPosn_flg]  "VTQD_LowBPSPosn_flg"
  Equal28/1 -> Switch9/2
  [VVMC_EstSlope_Deg] -> MTQD_CreepBPSDisPosn_Y_pct/1
  [VTQD_GearActualPosn_enum] -> Equal28/1
  Constant42/1 -> Equal27/2
  Switch8/1 -> Equal5/2
  [VVMC_EstSlope_Deg] -> MTQD_CreepBPSEnPosnR_Y_pct/1
  MTQD_CreepBPSEnPosn_Y_pct/1 -> Switch8/3  "VTQD_CreepBPSEnPosn_pct"
  MTQD_CreepBPSDisPosnR_Y_pct/1 -> Switch9/1  "VTQD_CreepBPSDisPosnR_pct"
  [VTQD_GearActualPosn_enum] -> Equal27/1
  MTQD_CreepBPSEnPosnR_Y_pct/1 -> Switch8/1  "VTQD_CreepBPSEnPosnR_pct"
  [VTQD_ActBPSPosn_pct] -> Equal5/1
  [VVMC_EstSlope_Deg] -> MTQD_CreepBPSEnPosn_Y_pct/1
  [VTQD_PreLoadPreEn_flg] -> NOT11/1
  [VINP_VehSpeed_kph] -> MTQD_CreepPreloadTime_Y_s/1
  Delay/1 -> Switch10/1
  [VTQD_CreepEnable_flg] -> Delay1/1
  Delay1/1 -> Switch10/2
  MTQD_CreepPreloadTime_Y_s/1 -> Switch10/3  "VTQD_CreepPreloadSetTime_s"
  Switch10/1 -> Delay/1, Relational Operator/2, Timer/4
  MTQD_CreepPterm_Y_c/1 -> [VTQD_CreepPterm_c]  "VTQD_CreepPterm_c"
  Add/1 -> [VTQD_CreepErrSpd_kph]  "VTQD_CreepErrSpd_kph"
  [VINP_VehSpeed_kph] -> MTQD_CreepPrelaodTq_Z_Nm/2
  [VVMC_EstSlope_Deg] -> MTQD_CreepBaseTqR_Z_Nm/1
  MTQD_CreepBaseTqD_Z_Nm/1 -> VTQD_CreepBaseTqD_Nm/1, [VTQD_CreepBaseTqD_Nm]  "VTQD_CreepBaseTqD_Nm"
  [VTQD_VehActSpd_kph] -> MTQD_CreepBaseTqD_Z_Nm/2
  MTQD_CreepDeltaTq_Y_Nm/1 -> [VTQD_CreepDeltaTq_Nm]  "VTQD_CreepDeltaTq_Nm"
  [VTQD_CreepErrSpd_kph] -> MTQD_CreepPterm_Y_c/1
  [VTQD_VehActSpd_kph] -> Add/2
  [VTQD_VehActSpd_kph] -> MTQD_CreepBaseTqR_Z_Nm/2
  [VTQD_CreepPreloadTime_s] -> MTQD_CreepPrelaodTq_Z_Nm/1
  MTQD_CreepBaseTqR_Z_Nm/1 -> VTQD_CreepBaseTqR_Nm/1, [VTQD_CreepBaseTqR_Nm]  "VTQD_CreepBaseTqR_Nm"
  [VTQD_CreepFinalSpd_kph] -> Add/1
  [VVMC_EstSlope_Deg] -> MTQD_CreepBaseTqD_Z_Nm/1
  MTQD_CreepPrelaodTq_Z_Nm/1 -> [VTQD_CreepPreloadTq_Nm]  "VTQD_CreepPreloadTq_Nm"
  MTQD_CreepProtTq_Y_Nm/1 -> [VTQD_CreepProtTq_Nm]  "VTQD_CreepProtTq_Nm"
  [VTQD_CreepErrSpd_kph] -> MTQD_CreepDeltaTq_Y_Nm/1
  [VVMC_EstSlope_Deg] -> MTQD_CreepProtTq_Y_Nm/1
  [VTQD_GearActualPosn_enum] -> Detect Change/1
  Constant46/1 -> Switch6/3
  [VTQD_LowBPSPosn_flg] -> NOT12/1
  [VTQD_HighBPSPosn_flg] -> NOT13/1
  NOT12/1 -> AND6/1
  NOT13/1 -> AND6/2
  Constant55/1 -> Equal34/2
  [VINP_EPBSta_enum] -> Equal34/1
  Constant16/1 -> Product1/3
  Constant19/1 -> Product1/4
  [VTQD_VehActSpdGain_gain] -> Product/1
  Constant47/1 -> FirstOrderFilter/3
  Switch11/1 -> VTQD_VehActSpd_kph/1, [VTQD_VehActSpd_kph]  "VTQD_VehActSpd_kph"
  FirstOrderFilter/1 -> [VTQD_RPM2VehSpd_kph]  "VTQD_RPM2VehSpd_kph"
  Product1/1 -> FirstOrderFilter/1
  Relay1/1 -> Switch11/2
  [VTQD_RPM2VehSpd_kph] -> Switch11/1
  Product/1 -> Switch11/3
  [VINP_VehSpeed_kph] -> Product/2
  Constant14/1 -> Product1/2
  [task_time_s] -> FirstOrderFilter/2
  [VINP_VehSpeed_kph] -> Relay1/1
  [VTQD_TqTargetShaftSpd_rpm] -> Product1/1
  Constant49/1 -> [VTQD_CreepTargetSpdD_kph]  "VTQD_CreepTargetSpdD_kph"
  Add2/1 -> Saturation Dynamic/2
  Constant22/1 -> Saturation Dynamic/3
  Constant57/1 -> Saturation Dynamic/1  "VTQD_CreepUpLimitTq_Nm"
  Saturation Dynamic/1 -> Switch/1
  VINP_EPBSta_enum/1 -> [VINP_EPBSta_enum]
  VTQD_TqTargetShaftSpd_rpm/1 -> [VTQD_TqTargetShaftSpd_rpm]
  NOT1/1 -> AND1/2
  GreaterThan/1 -> AND1/1
  [VTQD_VehActSpd_kph] -> MTQD_CreepIterm_Z_Nm/1
  MTQD_CreepIterm_Z_Nm/1 -> [VTQD_CreepIterm_c]  "VTQD_CreepIterm_c"
  [VTQD_CreepErrSpd_kph] -> MTQD_CreepIterm_Z_Nm/2
  Equal14/1 -> Logical Operator3/8
  NOT11/1 -> Logical Operator3/9
  OR/1 -> OR1/5
  [VTQD_RBCActive_flg] -> OR1/6
  Equal18/1 -> OR1/7
  Detect Change/1 -> OR1/8
  Equal34/1 -> OR1/9

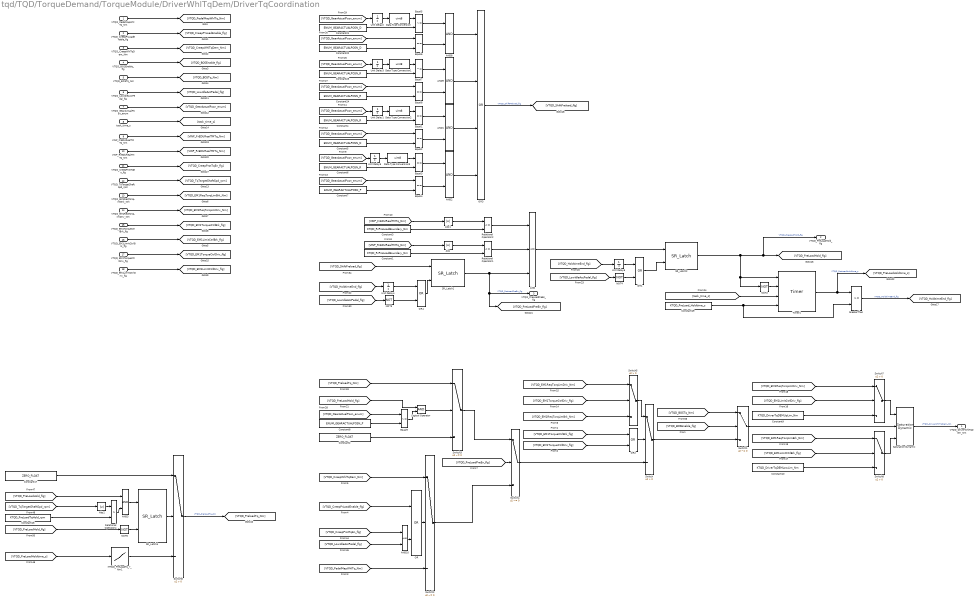
== system tqd/TQD/TorqueDemand/TorqueModule/DriverWhlTqDem/DriverTqCoordination ==
  VTQD_PedalMapWhlTq_Nm : Inport
  VTQD_CreepPrLoadEnable_flg : Inport  Port=2
  VTQD_CreepWhlTqDem_Nm : Inport  Port=3
  VTQD_BOSEnable_flg : Inport  Port=4
  VTQD_BOSTq_Nm : Inport  Port=5
  VTQD_LowIdleAccPedal_flg : Inport  Port=6
  VTQD_GearActualPosn_enum : Inport  Port=7
  task_time_s : Inport  Port=8
  VINP_FrEDURealTMTq_Nm : Inport  Port=9
  VINP_RrEDURealTMTq_Nm : Inport  Port=10
  VTQD_CreepProtTqEn_flg : Inport  Port=11
  VTQD_TqTargetShaftSpd_rpm : Inport  Port=12
  VTQD_EM1ReqTorqLimBrk_Nm : Inport  Port=13
  VTQD_EM1ReqTorqLimDriv_Nm : Inport  Port=14
  VTQD_EM1TorqueCtrlBrk_flg : Inport  Port=15
  VTQD_EM1LimitCtrlBrk_flg : Inport  Port=16
  VTQD_EM1TorqueCtrlDriv_flg : Inport  Port=17
  VTQD_EM1LimitCtrlDriv_flg : Inport  Port=18
  AND : Logic  Inputs=3  AllPortsSameDT=off  OutDataTypeStr=boolean
  AND{1..3,8..10} (6 alike) : Logic  AllPortsSameDT=off  OutDataTypeStr=boolean
  Abs : Abs
  Abs1 : Abs
  Abs2 : Abs
  Constant1 : Constant  Value=KTQD_RrPreLoadBoundary_Nm
  Constant10 : Constant  Value=KTQD_DriverTqDEMLowLim_Nm
  Constant16 : Constant  Value=KTQD_PreLoadTqHold_rpm
  Constant17 : Constant  Value=ZERO_FLOAT
  Constant19 : Constant  Value=KTQD_PreLoad_Holdtime_s
  Constant2 : Constant  Value=ZERO_FLOAT
  Constant21 : Constant  Value=ENUM_GEARACTUALPOSN_D
  Constant22 : Constant  Value=ENUM_GEARACTUALPOSN_D
  Constant{4,6,23..24} (4 alike) : Constant  Value=ENUM_GEARACTUALPOSN_R
  Constant3 : Constant  Value=KTQD_RrPreLoadBoundary_Nm
  Constant5 : Constant  Value=ENUM_GEARACTUALPOSN_N
  Constant7 : Constant  Value=ENUM_GEARACTUALPOSN_P
  Constant8 : Constant  Value=ENUM_GEARACTUALPOSN_P
  Constant9 : Constant  Value=KTQD_DriverTqDEMUpLim_Nm
  Data Type Conversion{,1..3} (4 alike) : DataTypeConversion  OutDataTypeStr=uint8
  Equal{1..4,6,8} (6 alike) : RelationalOperator  Operator===  OutDataTypeStr=boolean  RndMeth=Simplest
  Equal5 : RelationalOperator  Operator=~=  OutDataTypeStr=boolean  RndMeth=Simplest
  Equal7 : RelationalOperator  Operator=~=  OutDataTypeStr=boolean  RndMeth=Simplest
  Equal9 : RelationalOperator  Operator=~=  OutDataTypeStr=boolean  RndMeth=Simplest
  GreaterThan : RelationalOperator  OutDataTypeStr=boolean  RndMeth=Simplest
  Logical Operator : Logic  AllPortsSameDT=off  OutDataTypeStr=boolean
  MTQD_PreLoadTq_Y_Nm1 : Lookup_n-D  NumberOfTableDimensions=1  BreakpointsForDimension1=ATQD_PreLoadTq_X_s  Table=MTQD_PreLoadTq_Y_Nm  ExtrapMethod=Clip  InternalRulePriority=Speed  RndMeth=Simplest  InputSameDT=on
  NOT{2..4,6} (4 alike) : Logic  Operator=NOT  AllPortsSameDT=off  OutDataTypeStr=boolean
  OR{,1..2,4} (4 alike) : Logic  Operator=OR  AllPortsSameDT=off  OutDataTypeStr=boolean
  OR3 : Logic  Operator=OR  Inputs=4  AllPortsSameDT=off  OutDataTypeStr=boolean
  Relational Operator1 : RelationalOperator  Operator=<=  OutDataTypeStr=boolean  RndMeth=Simplest
  Relational Operator2 : RelationalOperator  Operator=<=  OutDataTypeStr=boolean  RndMeth=Simplest
  Relational Operator4 : RelationalOperator  Operator=>  OutDataTypeStr=boolean  RndMeth=Simplest
  SR_Latch1 : hcu_lib/Basic_Blocks/SR_Latch
  SR_Latch2 : hcu_lib/Basic_Blocks/SR_Latch
  SR_Latch4 : hcu_lib/Basic_Blocks/SR_Latch
  Saturation Dynamic : simulink/Discontinuities/Saturation Dynamic  OutMin=[]  OutMax=[]  OutDataTypeStr=Inherit: Same as second input  OutDataType=fixdt(1, 16)  OutScaling=2^-10  DoSatur=off
  Switch{,5..8} (5 alike) : Switch  Criteria=u2 > Threshold
  Switch{1..4} (4 alike) : Switch  Criteria=u2 ~= 0
      Switch1 settings: AttributesFormatString=<%<Criteria>>
      Switch2 settings: AttributesFormatString=<%<Criteria>>
  Timer1 : hcu_lib/Basic_Blocks/Timer
  Unit Delay{1..6} (6 alike) : UnitDelay  SampleTime=-1  HasFrameUpgradeWarning=on
  VTQD_DriverWhlTqDem_Nm : Outport
  VTQD_PreLoadHold_flg : Outport  Port=2
  VTQD_PreLoadPreEn_flg : Outport  Port=3
  wires:
  VTQD_PedalMapWhlTq_Nm/1 -> [VTQD_PedalMapWhlTq_Nm]
  VTQD_CreepPrLoadEnable_flg/1 -> [VTQD_CreepPrLoadEnable_flg]
  VTQD_CreepWhlTqDem_Nm/1 -> [VTQD_CreepWhlTqDem_Nm]
  VTQD_BOSEnable_flg/1 -> [VTQD_BOSEnable_flg]
  VTQD_BOSTq_Nm/1 -> [VTQD_BOSTq_Nm]
  [VTQD_BOSEnable_flg] -> Switch1/2
  [VTQD_PedalMapWhlTq_Nm] -> Switch2/3
  [VTQD_CreepWhlTqDem_Nm] -> Switch2/1
  VTQD_LowIdleAccPedal_flg/1 -> [VTQD_LowIdleAccPedal_flg]
  VTQD_GearActualPosn_enum/1 -> [VTQD_GearActualPosn_enum]
  task_time_s/1 -> [task_time_s]
  Timer1/1 -> [VTQD_PreLoadHoldtime_s], GreaterThan/1  "VTQD_PreLoadHoldtime_s"
  GreaterThan/1 -> [VTQD_HoldtimeEnd_flg]  "VTQD_HoldtimeEnd_flg"
  [VTQD_PreLoadPreEn_flg] -> Switch4/2
  [VTQD_HoldtimeEnd_flg] -> Unit Delay4/1
  Constant19/1 -> GreaterThan/2, Timer1/4
  [task_time_s] -> Timer1/3
  Unit Delay2/1 -> Data Type Conversion/1
  [VTQD_GearActualPosn_enum] -> Unit Delay2/1
  Constant23/1 -> Equal7/2
  [VTQD_GearActualPosn_enum] -> Equal8/1
  Equal5/1 -> AND8/1
  AND9/1 -> OR3/2
  Constant21/1 -> Equal5/2
  Constant24/1 -> Equal8/2
  Unit Delay3/1 -> Data Type Conversion1/1
  Constant22/1 -> Equal6/2
  AND8/1 -> OR3/1
  [VTQD_GearActualPosn_enum] -> Unit Delay3/1
  [VTQD_GearActualPosn_enum] -> Equal6/1
  Equal6/1 -> AND8/2
  Equal8/1 -> AND9/2
  OR3/1 -> [VTQD_ShiftPreload_flg]  "VTQD_ShiftPreload_flg"
  Equal7/1 -> AND9/1
  NOT2/1 -> Timer1/2
  Unit Delay4/1 -> OR4/1
  OR4/1 -> SR_Latch1/2
  Switch2/1 -> Switch4/3
  [VTQD_LowIdleAccPedal_flg] -> NOT3/1
  NOT3/1 -> OR4/2
  VINP_FrEDURealTMTq_Nm/1 -> [VINP_FrEDURealTMTq_Nm]
  VINP_RrEDURealTMTq_Nm/1 -> [VINP_RrEDURealTMTq_Nm]
  [VTQD_GearActualPosn_enum] -> Equal2/1
  Constant5/1 -> Equal2/2
  Equal2/1 -> AND1/2
  Equal1/1 -> AND1/1
  Constant4/1 -> Equal1/2
  AND1/1 -> OR3/3
  [VTQD_GearActualPosn_enum] -> Unit Delay1/1
  Unit Delay1/1 -> Data Type Conversion2/1
  Constant3/1 -> Relational Operator2/2
  Relational Operator2/1 -> AND/1
  Constant1/1 -> Relational Operator1/2
  Abs1/1 -> Relational Operator2/1
  Relational Operator1/1 -> AND/2
  Abs/1 -> Relational Operator1/1
  [VINP_RrEDURealTMTq_Nm] -> Abs/1
  [VINP_FrEDURealTMTq_Nm] -> Abs1/1
  SR_Latch1/1 -> VTQD_PreLoadPreEn_flg/1, [VTQD_PreLoadPreEn_flg], AND/3  "VTQD_PreLoadPreEn_flg"
  Switch3/1 -> Switch4/1
  Constant2/1 -> Switch3/3
  Unit Delay5/1 -> Data Type Conversion3/1
  [VTQD_GearActualPosn_enum] -> Unit Delay5/1
  Constant6/1 -> Equal3/2
  Equal3/1 -> AND2/1
  Equal4/1 -> AND2/2
  Constant7/1 -> Equal4/2
  [VTQD_GearActualPosn_enum] -> Equal4/1
  AND2/1 -> OR3/4
  AND/1 -> SR_Latch2/1
  NOT4/1 -> OR1/2
  [VTQD_LowIdleAccPedal_flg] -> NOT4/1
  Unit Delay6/1 -> OR1/1
  [VTQD_HoldtimeEnd_flg] -> Unit Delay6/1
  OR1/1 -> SR_Latch2/2
  [VTQD_GearActualPosn_enum] -> Equal9/1
  Constant8/1 -> Equal9/2
  Logical Operator/1 -> Switch3/2
  [VTQD_PreLoadHold_flg] -> Logical Operator/1
  Equal9/1 -> Logical Operator/2
  SR_Latch2/1 -> VTQD_PreLoadHold_flg/1, [VTQD_PreLoadHold_flg], NOT2/1, Timer1/1  "VTQD_PreLoadHold_flg"
  [VTQD_PreloadTq_Nm] -> Switch3/1
  OR/1 -> Switch2/2
  [VTQD_CreepPrLoadEnable_flg] -> OR/1
  VTQD_CreepProtTqEn_flg/1 -> [VTQD_CreepProtTqEn_flg]
  [VTQD_CreepProtTqEn_flg] -> AND10/1
  [VTQD_LowIdleAccPedal_flg] -> AND10/2
  AND10/1 -> OR/2
  [VTQD_PreLoadHold_flg] -> AND3/1
  Constant17/1 -> Switch6/1
  Abs2/1 -> Relational Operator4/1
  [VTQD_PreLoadHold_flg] -> NOT6/1
  [VTQD_TqTargetShaftSpd_rpm] -> Abs2/1
  Constant16/1 -> Relational Operator4/2
  NOT6/1 -> SR_Latch4/2
  Switch6/1 -> [VTQD_PreloadTq_Nm]  "VTQD_PreloadTq_Nm"
  SR_Latch4/1 -> Switch6/2
  MTQD_PreLoadTq_Y_Nm1/1 -> Switch6/3
  Relational Operator4/1 -> AND3/2
  AND3/1 -> SR_Latch4/1
  [VTQD_PreLoadHoldtime_s] -> MTQD_PreLoadTq_Y_Nm1/1
  VTQD_TqTargetShaftSpd_rpm/1 -> [VTQD_TqTargetShaftSpd_rpm]
  [VTQD_BOSTq_Nm] -> Switch1/1
  [VTQD_ShiftPreload_flg] -> SR_Latch1/1
  Data Type Conversion/1 -> Equal5/1
  Data Type Conversion1/1 -> Equal7/1
  Data Type Conversion2/1 -> Equal1/1
  Data Type Conversion3/1 -> Equal3/1
  VTQD_EM1LimitCtrlBrk_flg/1 -> [VTQD_EM1LimitCtrlBrk_flg]
  VTQD_EM1TorqueCtrlBrk_flg/1 -> [VTQD_EM1TorqueCtrlBrk_flg]
  VTQD_EM1ReqTorqLimDriv_Nm/1 -> [VTQD_EM1ReqTorqLimDriv_Nm]
  VTQD_EM1ReqTorqLimBrk_Nm/1 -> [VTQD_EM1ReqTorqLimBrk_Nm]
  VTQD_EM1TorqueCtrlDriv_flg/1 -> [VTQD_EM1TorqueCtrlDriv_flg]
  VTQD_EM1LimitCtrlDriv_flg/1 -> [VTQD_EM1LimitCtrlDriv_flg]
  Switch4/1 -> Switch/3
  OR2/1 -> Switch/2
  [VTQD_EM1TorqueCtrlBrk_flg] -> OR2/1
  [VTQD_EM1TorqueCtrlDriv_flg] -> OR2/2
  Switch5/1 -> Switch/1
  [VTQD_EM1ReqTorqLimBrk_Nm] -> Switch5/3
  [VTQD_EM1TorqueCtrlDriv_flg] -> Switch5/2
  [VTQD_EM1ReqTorqLimDriv_Nm] -> Switch5/1
  Switch/1 -> Switch1/3
  Saturation Dynamic/1 -> VTQD_DriverWhlTqDem_Nm/1  "VTQD_DriverWhlTqDem_Nm"
  Switch1/1 -> Saturation Dynamic/2
  Switch7/1 -> Saturation Dynamic/1
  Switch8/1 -> Saturation Dynamic/3
  [VTQD_EM1LimitCtrlBrk_flg] -> Switch8/2
  [VTQD_EM1LimitCtrlDriv_flg] -> Switch7/2
  Constant10/1 -> Switch8/3
  Constant9/1 -> Switch7/3
  [VTQD_EM1ReqTorqLimDriv_Nm] -> Switch7/1
  [VTQD_EM1ReqTorqLimBrk_Nm] -> Switch8/1

== system tqd/TQD/TorqueDemand/TorqueModule/DriverWhlTqDem/PedalMapWhlTq ==
  VTQD_GearActualPosn_enum : Inport
  VTQD_ActAPSPosn_pct : Inport  Port=2
  VTQD_TqTargetShaftSpd_rpm : Inport  Port=3
  VTQD_LimpHomeAct_flg : Inport  Port=4
  VTQD_EVDriveMode_enum : Inport  Port=5
  VTQD_RegenMode_enum : Inport  Port=6
  VTQD_RollRegenDisableReq_flg : Inport  Port=7
  VINP_HSAActive_flg : Inport  Port=8
  VVMC_EstSlope_Deg : Inport  Port=9
  AND : Logic  AllPortsSameDT=off  OutDataTypeStr=boolean
  Abs : Abs
  Abs1 : Abs
  Constant10 : Constant  Value=KTQD_ClimbMin_rpm
  Constant11 : Constant  Value=KTQD_PedalMapRDCUpLim_Nm
  Constant12 : Constant  Value=KTQD_PedalMapRDCLowLim_Nm
  Constant5 : Constant  Value=KTQD_PedalMapClimbLowLim_Nm
  GearShiftCheck : If  IfExpression=u1~= 0
  LHM : Subsystem  TreatAsAtomicUnit=on
  MTQD_PedalMapClimbUpLim_Z_Nm : Lookup_n-D  BreakpointsForDimension1=ATQD_PedalMapClimbUpLim_Y_Deg  BreakpointsForDimension2=ATQD_PedalMapClimbUpLim_X_rpm  Table=MTQD_PedalMapClimbUpLim_Z_Nm  ExtrapMethod=Clip  InternalRulePriority=Speed  RndMeth=Simplest  InputSameDT=on
      settings: InputPortMap=u0,u1
  Merge : Merge
  NOT : Logic  Operator=NOT  AllPortsSameDT=off  OutDataTypeStr=boolean
  NoLHM : Subsystem  TreatAsAtomicUnit=on
  Relational Operator : RelationalOperator  Operator=<=  OutDataTypeStr=boolean  RndMeth=Simplest
  SR_Latch : hcu_lib/Basic_Blocks/SR_Latch
  Saturation Dynamic : simulink/Discontinuities/Saturation Dynamic  OutMin=[]  OutMax=[]  OutDataTypeStr=Inherit: Same as second input  OutDataType=fixdt(1, 16)  OutScaling=2^-10  DoSatur=off
  Saturation Dynamic1 : simulink/Discontinuities/Saturation Dynamic  OutMin=[]  OutMax=[]  OutDataTypeStr=Inherit: Same as second input  OutDataType=fixdt(1, 16)  OutScaling=2^-10  DoSatur=off
  Switch3 : Switch  Criteria=u2 ~= 0
  Switch4 : Switch  Criteria=u2 ~= 0
  VTQD_PedalMapWhlTq_Nm : Outport
  wires:
  [VTQD_GearActualPosn_enum] -> LHM/3(VTQD_GearActualPosn_enum)
  LHM/1(VTQD_PedalMapWhlTqLHM_Nm) -> Merge/1
  NoLHM/1(VTQD_PedalMapWhlTqNoLHM_Nm) -> Merge/2
  [VTQD_EVDriveMode_enum] -> NoLHM/5(VTQD_EVDriveMode_enum)
  [VTQD_GearActualPosn_enum] -> NoLHM/4(VTQD_GearActualPosn_enum)
  GearShiftCheck/2 -> NoLHM/Action
  GearShiftCheck/1 -> LHM/Action
  [VTQD_LimpHomeAct_flg] -> GearShiftCheck/1
  VTQD_RegenMode_enum/1 -> [VTQD_RegenMode_enum]
  VTQD_ActAPSPosn_pct/1 -> [VTQD_ActAPSPosn_pct]
  VTQD_EVDriveMode_enum/1 -> [VTQD_EVDriveMode_enum]
  VTQD_LimpHomeAct_flg/1 -> [VTQD_LimpHomeAct_flg]
  VTQD_GearActualPosn_enum/1 -> [VTQD_GearActualPosn_enum]
  VTQD_TqTargetShaftSpd_rpm/1 -> [VTQD_TqTargetShaftSpd_rpm]
  [VTQD_TqTargetShaftSpd_rpm] -> NoLHM/2(VTQD_TqTargetShaftSpd_rpm)
  [VTQD_RegenMode_enum] -> NoLHM/3(VTQD_RegenMode_enum)
  [VTQD_ActAPSPosn_pct] -> NoLHM/1(VTQD_ActAPSPosn_pct)
  [VTQD_ActAPSPosn_pct] -> LHM/1(VTQD_ActAPSPosn_pct)
  [VTQD_TqTargetShaftSpd_rpm] -> LHM/2(VTQD_TqTargetShaftSpd_rpm)
  VTQD_RollRegenDisableReq_flg/1 -> [VTQD_RollRegenDisableReq_flg]
  VINP_HSAActive_flg/1 -> [VINP_HSAActive_flg]
  Switch3/1 -> Switch4/3
  [VTQD_TqTargetShaftSpd_rpm] -> Abs/1
  Constant5/1 -> Saturation Dynamic/3
  SR_Latch/1 -> AND/1
  Relational Operator/1 -> AND/2, NOT/1
  Constant10/1 -> Relational Operator/2
  Constant12/1 -> Saturation Dynamic1/3
  Saturation Dynamic1/1 -> Switch4/1
  Saturation Dynamic/1 -> Switch3/1
  Abs/1 -> Relational Operator/1
  Abs1/1 -> MTQD_PedalMapClimbUpLim_Z_Nm/2
  [VTQD_TqTargetShaftSpd_rpm] -> Abs1/1
  AND/1 -> Switch3/2  "VTQD_ActHSAActive_flg"
  [VVMC_EstSlope_Deg] -> MTQD_PedalMapClimbUpLim_Z_Nm/1
  NOT/1 -> SR_Latch/2
  MTQD_PedalMapClimbUpLim_Z_Nm/1 -> Saturation Dynamic/1  "VTQD_PedalMapClimbUpLim_Nm"
  Constant11/1 -> Saturation Dynamic1/1
  [VTQD_RollRegenDisableReq_flg] -> Switch4/2
  VVMC_EstSlope_Deg/1 -> [VVMC_EstSlope_Deg]
  Merge/1 -> Switch3/3, Saturation Dynamic/2, Saturation Dynamic1/2  "VTQD_OrigPedalMapWhlTq_Nm"
  Switch4/1 -> VTQD_PedalMapWhlTq_Nm/1  "VTQD_PedalMapWhlTq_Nm"
  [VINP_HSAActive_flg] -> SR_Latch/1
